simulink model "Ond_MLI_1"  (R2020a)
settings: Solver=VariableStepAuto  StartTime=0.0  StopTime=1  FixedStep=0.0001  RelTol=1e-3  EnableMultiTasking=on
InitFcn:
  | E=150;
  | V=220;
  | fs=50;
  | A=1;
  | 
  | Teta_0=0;
  | Cr=0;
  | Rr=3.805;
  | J=0.031;
  | f=0;
  | p=2;
  | Rs=4.85;
  | M=0.258;
  | Ls=0.274;
  | Lr=0.274;
  | R=[Rs 0 0 0;0 Rs 0 0;0 0 Rs 0;0 0 0 Rs];
  | L=[Ls 0 M 0;0 Ls 0 M;M 0 Lr 0;0 M 0 Lr];
  | A1=[0 -Ls 0 -M;Ls 0 M 0;0 0 0 0;0 0 0 0];
  | A2=[0 0 0 0;0 0 0 0;0 -M 0 -Lr;M 0 Lr 0];
undefined symbols (not defined in the file): Vp
libraries: powerlib x11, simulink x2, powerlib_meascontrol x2
settings Model: SimulationMode=accelerator  Creator=SINA  LastModifiedBy=ABO-CHIFA
settings DataIOCC: ReturnWorkspaceOutputs=off
settings OptimizationCC: LifeSpan=inf
settings DebuggingCC: SFUnexpectedBacktrackingDiag=warning  SFNoUnconditionalDefaultTransitionDiag=warning  ArithmeticOperatorsInVariantConditions=warning
settings SFSimCC: SimUseLocalCustomCode=off  CustomCodeUndefinedFunction=UseInterfaceOnly
settings RTWCC: RTWUseLocalCustomCode=off
settings CodeAppCC: StateflowObjectComments=on
settings GRTTargetCC: TargetLangStandard=C89/C90 (ANSI)
settings ConfigComp: CovMetricSettings=dw  CovHtmlReporting=on  CovSaveCumulativeToWorkspaceVar=on  CovSaveSingleToWorkspaceVar=on  CovExternalEMLEnable=off
settings SimscapeCC: SimscapeNormalizeSystem=off

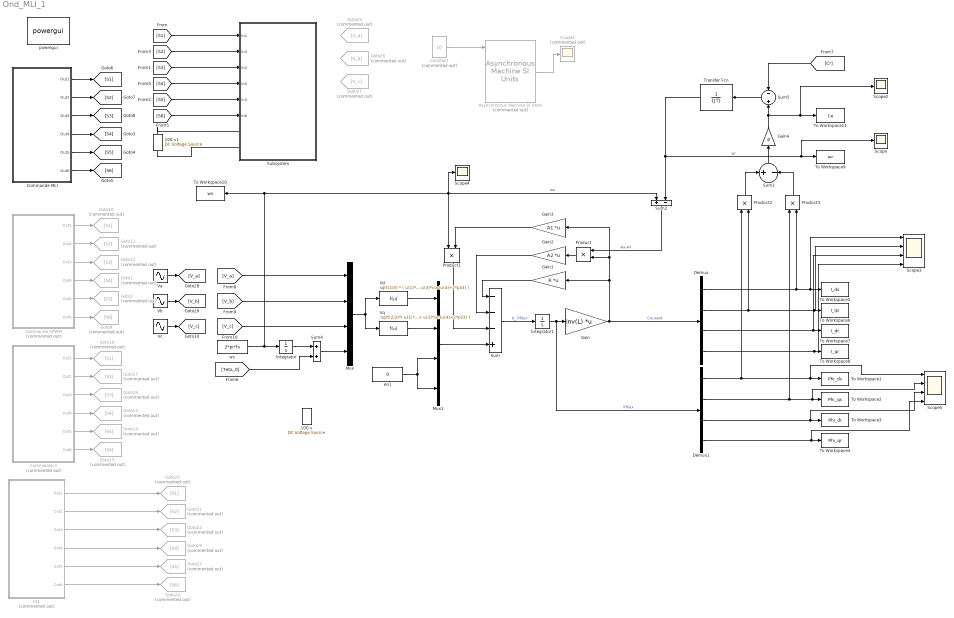
== system Ond_MLI_1 ==
  100 v : powerlib/Electrical Sources/DC Voltage Source  Amplitude=E  Measurements=Voltage
  100 v1 : powerlib/Electrical Sources/DC Voltage Source  Amplitude=E  Measurements=Voltage
  Asynchronous Machine SI Units : powerlib/Machines/Asynchronous Machine SI Units  Commented=on  RotorType=Squirrel-cage  PresetModel="15:  5.4 HP (4KW)   400 V  50Hz 1430 RPM"  MechanicalLoad=Torque Tm  ShowDetailedParameters=on  ReferenceFrame=Rotor  Units=SI  MeasurementBus=off  NominalParameters=[4000 400 50]  Stator=[1.405 0.005839]  Rotor=[1.395 0.005839]  Cage1=[0.4155 0.002066]  Cage2=[0.4168 0.0003495]  Lm=0.1722  Mechanical=[0.0131 0.002985 2]  PolePairs=2  InitialConditions=[1 0 0 0 0 0 0 0]  SimulateSaturation=off  Saturation=[14.03593122, 27.81365428, 53.79336849, 72.68890987, 97.98006896, 148.6815601, 215.7428561, 302.9841135, 428.7778367 ; 230, 322, 414, 460, 506, 552, 598, 644, 690]  LoadFlowParameters=1492000  TsPowergui=0  TsBlock=-1  IterativeModel=Trapezoidal non iterative  IterativeDiscreteModel=Trapezoidal non iterative  Pmec=1.492e+006
  "Commande 3 " : Subsystem  Commented=on
  "Commande MLI " : Subsystem
  "Commande SPWM " : Subsystem  Commented=on
  Constant : Constant  Commented=on  Value=10
  Demux : Demux
  Demux1 : Demux
  Gain : Gain  Gain=inv(L)  Multiplication=Matrix(K*u)
  Gain1 : Gain  Gain=R  Multiplication=Matrix(K*u)
  Gain2 : Gain  Gain=A2  Multiplication=Matrix(K*u)
  Gain3 : Gain  Gain=A1  Multiplication=Matrix(K*u)
  Gain4 : Gain  Gain=p
  Goto1 : Goto  Commented=on  GotoTag=S4
  Goto10 : Goto  Commented=on  GotoTag=S1
  Goto11 : Goto  Commented=on  GotoTag=S2
  Goto12 : Goto  Commented=on  GotoTag=S3
  Goto13 : Goto  Commented=on  GotoTag=S4
  Goto14 : Goto  Commented=on  GotoTag=S5
  Goto15 : Goto  Commented=on  GotoTag=S6
  Goto16 : Goto  Commented=on  GotoTag=S1
  Goto17 : Goto  Commented=on  GotoTag=S2
  Goto18 : Goto  Commented=on  GotoTag=S3
  Goto19 : Goto  Commented=on  GotoTag=S4
  Goto2 : Goto  Commented=on  GotoTag=S5
  Goto20 : Goto  Commented=on  GotoTag=S1
  Goto21 : Goto  Commented=on  GotoTag=S2
  Goto22 : Goto  Commented=on  GotoTag=S3
  Goto23 : Goto  Commented=on  GotoTag=S5
  Goto24 : Goto  Commented=on  GotoTag=S6
  Goto25 : Goto  Commented=on  GotoTag=V_a
  Goto26 : Goto  Commented=on  GotoTag=V_b
  Goto27 : Goto  Commented=on  GotoTag=V_c
  Goto9 : Goto  Commented=on  GotoTag=S6
  Integrator : Integrator
  Integrator1 : Integrator
  Mux : Mux
  Mux1 : Mux
  Product{,1..3} (4 alike) : Product
  Scope : Scope
  Scope1 : Scope  Commented=on
  Scope2 : Scope
  Scope3 : Scope  NumInputPorts=4
  Scope4 : Scope
  Scope5 : Scope  NumInputPorts=4
  Subsystem : Subsystem
  Sum : Sum  Inputs=---+
  Sum1 : Sum  Inputs=+-
  Sum2 : Sum  Inputs=+-
  Sum4 : Sum
  Sum5 : Sum  Inputs=-+
  To Workspace1 : ToWorkspace  VariableName=Phi_ds  SampleTime=-1
  To Workspace10 : ToWorkspace  VariableName=ws  SampleTime=-1
  To Workspace11 : ToWorkspace  VariableName=Ce  SampleTime=-1
  To Workspace2 : ToWorkspace  VariableName=Phi_qs  SampleTime=-1
  To Workspace3 : ToWorkspace  VariableName=Phi_dr  SampleTime=-1
  To Workspace4 : ToWorkspace  VariableName=Phi_qr  SampleTime=-1
  To Workspace5 : ToWorkspace  VariableName=I_ds  SampleTime=-1
  To Workspace6 : ToWorkspace  VariableName=I_qs  SampleTime=-1
  To Workspace7 : ToWorkspace  VariableName=I_dr  SampleTime=-1
  To Workspace8 : ToWorkspace  VariableName=I_qr  SampleTime=-1
  To Workspace9 : ToWorkspace  VariableName=wr  SampleTime=-1
  Transfer Fcn : TransferFcn  Denominator=[J f]
  Va : Sin  Amplitude=V*sqrt(2)  Frequency=2*pi*fs  SampleTime=0
  Vb : Sin  Amplitude=V*sqrt(2)  Frequency=2*pi*fs  Phase=-2*pi/3  SampleTime=0
  Vc : Sin  Amplitude=V*sqrt(2)  Frequency=2*pi*fs  Phase=2*pi/3  SampleTime=0
  Vd : Fcn  Expr="sqrt(2/3) * ( u(1)*cos(u(4))  + u(2)*cos(u(4)-2*pi/3) + u(3)*cos(u(4)+2*pi/3) )"
  Vq : Fcn  Expr="-sqrt(2/3)*( u(1)*sin(u(4))  + u(2)*sin(u(4)-2*pi/3) + u(3)*sin(u(4)+2*pi/3) )"
  powergui : powerlib/powergui  Priority=1  SimulationMode=Discrete  SampleTime=1e-6  frequency=60  Iterations=50  frequencyindice=0  Pbase=100e6  ErrMax=1e-4  UnitsV=kV  UnitsW=MW  buscounter=0  FunctionMessages=off  echomessages=off  EnableUseOfTLC=off  CurrentSourceSwitches=off  DisableSnubberDevices=off  DisableRonSwitches=off  DisableVfSwitches=off  DisplayEquations=off  AutomaticDiscreteSolvers=off  SolverType=Tustin/Backward Euler (TBE)  Interpol=off  ExternalGateDelay=off  methode=off  Ts=10  x0status=blocks  SPID=off  SwTol=0  HookPort=off  NonlinearTolerance=1e-4  nMaxIteration=100  ContinueOnMaxIteration=off  RestoreLinks=warning  ResistiveCurrentMeasurement=off  Frange=[0:2:500]  Ylog=off  Xlog=on  ShowGrid=off  save=off  variable=ZData  structure=0  ZoomFFT=off  StartTime=0.0  cycles=1  DisplayStyle=1  fundamental=60  FreqAxis=off  MaxFrequency=1000  frequencyindicesteady=1  RmsSteady=1  display=off
  "tri1 " : Subsystem  Commented=on
  ws : Constant  Value=2*pi*fs
  ws1 : Constant  Value=0
  wires:
  "Commande MLI "/4(Out4) -> [S4]
  "Commande MLI "/5(Out5) -> [S5]
  "Commande MLI "/6(Out6) -> [S6]
  "Commande MLI "/2(Out2) -> [S2]
  "Commande MLI "/1(Out1) -> [S1]
  "Commande MLI "/3(Out3) -> [S3]
  "Commande SPWM "/1(Out1) -> Goto10/1
  "Commande SPWM "/2(Out2) -> Goto11/1
  "Commande SPWM "/3(Out3) -> Goto12/1
  "Commande SPWM "/4(Out4) -> Goto1/1
  "Commande SPWM "/5(Out5) -> Goto2/1
  "Commande SPWM "/6(Out6) -> Goto9/1
  [S1] -> Subsystem/1(In1)
  [S3] -> Subsystem/3(In2)
  [S5] -> Subsystem/5(In3)
  [S2] -> Subsystem/2(In4)
  [S4] -> Subsystem/4(In5)
  [S6] -> Subsystem/6(In6)
  "Commande 3 "/1(Out1) -> Goto16/1
  "Commande 3 "/2(Out2) -> Goto17/1
  "Commande 3 "/3(Out3) -> Goto18/1
  "Commande 3 "/4(Out4) -> Goto13/1
  "Commande 3 "/5(Out5) -> Goto14/1
  "Commande 3 "/6(Out6) -> Goto15/1
  Asynchronous Machine SI Units/1 -> Scope1/1
  Constant/1 -> Asynchronous Machine SI Units/1
  "tri1 "/1(Out1) -> Goto20/1
  "tri1 "/2(Out2) -> Goto21/1
  "tri1 "/3(Out3) -> Goto22/1
  "tri1 "/4(Out4) -> Goto19/1
  "tri1 "/5(Out5) -> Goto23/1
  "tri1 "/6(Out6) -> Goto24/1
  ws/1 -> Sum2/1, Scope4/1, Product1/1, To Workspace10/1, Integrator/1  "ws"
  Mux/1 -> Vd/1, Vq/1
  Vd/1 -> Mux1/1
  Vq/1 -> Mux1/2
  ws1/1 -> Mux1/3, Mux1/4
  Sum/1 -> Integrator1/1  "d_ Phlux"
  Integrator1/1 -> Gain/1, Demux1/1  "Phlux"
  Gain/1 -> Demux/1, Gain3/1, Product/2, Gain1/1  "Courant"
  Product/1 -> Gain2/1
  Gain3/1 -> Product1/2
  Demux1/1 -> Product2/1, Scope5/1, To Workspace1/1
  Demux1/4 -> Scope5/4, To Workspace4/1
  Demux1/3 -> Scope5/3, To Workspace3/1
  Demux/4 -> Scope3/4, To Workspace8/1
  Demux/3 -> Scope3/3, To Workspace7/1
  Demux/2 -> Scope3/2, To Workspace6/1, Product2/2
  Demux/1 -> Scope3/1, To Workspace5/1, Product3/2
  Demux1/2 -> Product3/1, Scope5/2, To Workspace2/1
  Product2/1 -> Sum1/1
  Product3/1 -> Sum1/2
  Transfer Fcn/1 -> To Workspace9/1, Scope/1, Sum2/2  "wr"
  Sum2/1 -> Product/1  "ws-wr"
  Sum1/1 -> Gain4/1
  Integrator/1 -> Sum4/1
  Sum4/1 -> Mux/4
  [Teta_0] -> Sum4/2
  Sum5/1 -> Transfer Fcn/1
  Gain4/1 -> Sum5/2, To Workspace11/1, Scope2/1
  [V_a] -> Mux/1
  [V_b] -> Mux/2
  Vb/1 -> [V_b]
  Va/1 -> [V_a]
  Vc/1 -> [V_c]
  [V_c] -> Mux/3
  Mux1/1 -> Sum/4
  Product1/1 -> Sum/3
  Gain2/1 -> Sum/2
  Gain1/1 -> Sum/1
  [Cr] -> Sum5/1
  connections:
  100 v1/RConn1 -- Subsystem/LConn1
  100 v1/LConn1 -- Subsystem/LConn2

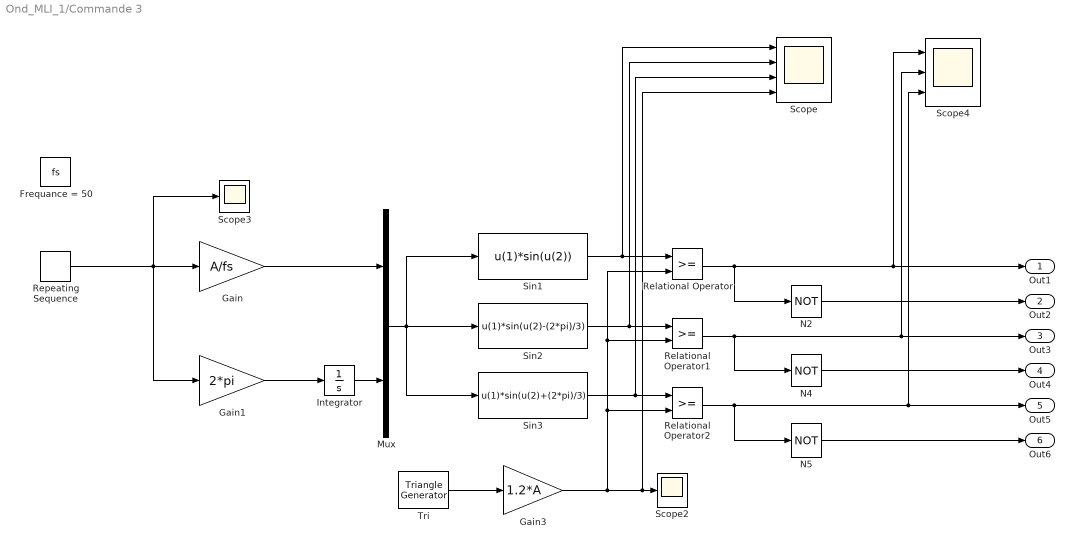
== system Ond_MLI_1/Commande 3  ==
  Frequance = 50 : Constant  Value=fs
  Gain : Gain  Gain=A/fs
  Gain1 : Gain  Gain=2*pi
  Gain3 : Gain  Gain=1.2*A
  Integrator : Integrator
  Mux : Mux  Inputs=2
  N2 : Logic  Operator=NOT  AllPortsSameDT=off  OutDataTypeStr=boolean
  N4 : Logic  Operator=NOT  AllPortsSameDT=off  OutDataTypeStr=boolean
  N5 : Logic  Operator=NOT  AllPortsSameDT=off  OutDataTypeStr=boolean
  Relational Operator : RelationalOperator  OutDataTypeStr=boolean  RndMeth=Nearest
  Relational Operator1 : RelationalOperator  OutDataTypeStr=boolean  RndMeth=Nearest
  Relational Operator2 : RelationalOperator  OutDataTypeStr=boolean  RndMeth=Nearest
  Repeating Sequence : simulink/Sources/Repeating Sequence  rep_seq_t=[0 0.1 10]  rep_seq_y=[0 fs fs]
  Scope : Scope  NumInputPorts=4
  Scope2 : Scope
  Scope3 : Scope
  Scope4 : Scope  NumInputPorts=3
  Sin1 : Fcn  Expr=u(1)*sin(u(2))
  Sin2 : Fcn  Expr=u(1)*sin(u(2)-(2*pi)/3)
  Sin3 : Fcn  Expr=u(1)*sin(u(2)+(2*pi)/3)
  Tri : powerlib_meascontrol/Pulse & Signal Generators/Triangle Generator  Freq=1e3  Phase=90  Ts=0
  Out1 : Outport
  Out2 : Outport  Port=2
  Out3 : Outport  Port=3
  Out4 : Outport  Port=4
  Out5 : Outport  Port=5
  Out6 : Outport  Port=6
  wires:
  Gain1/1 -> Integrator/1
  Integrator/1 -> Mux/2
  Gain/1 -> Mux/1
  Mux/1 -> Sin3/1, Sin2/1, Sin1/1
  N2/1 -> Out2/1
  N4/1 -> Out4/1
  Relational Operator2/1 -> N5/1, Out5/1, Scope4/3
  Gain3/1 -> Relational Operator2/2, Relational Operator1/2, Relational Operator/2, Scope2/1, Scope/4
  Tri/1 -> Gain3/1
  Sin1/1 -> Relational Operator/1, Scope/1
  Sin2/1 -> Relational Operator1/1, Scope/2
  Sin3/1 -> Relational Operator2/1, Scope/3
  N5/1 -> Out6/1
  Relational Operator1/1 -> N4/1, Out3/1, Scope4/2
  Relational Operator/1 -> Out1/1, Scope4/1, N2/1
  Repeating Sequence/1 -> Gain1/1, Scope3/1, Gain/1

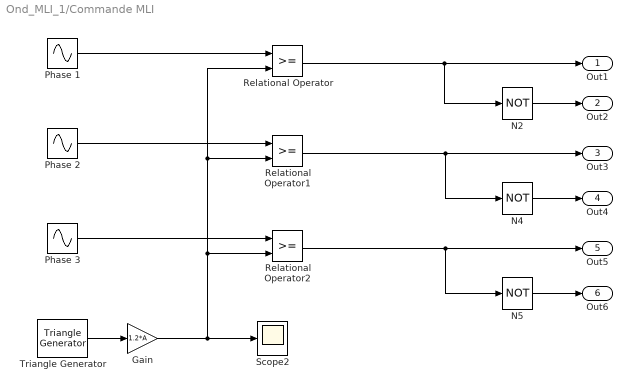
== system Ond_MLI_1/Commande MLI  ==
  Gain : Gain  Gain=1.2*A
  N2 : Logic  Operator=NOT  AllPortsSameDT=off  OutDataTypeStr=boolean
  N4 : Logic  Operator=NOT  AllPortsSameDT=off  OutDataTypeStr=boolean
  N5 : Logic  Operator=NOT  AllPortsSameDT=off  OutDataTypeStr=boolean
  "Phase 1 " : Sin  Amplitude=A  Frequency=2*pi*fs  SampleTime=0
  Phase 2 : Sin  Amplitude=A  Frequency=2*pi*fs  Phase=-2*pi/3  SampleTime=0
  Phase 3 : Sin  Amplitude=A  Frequency=2*pi*fs  Phase=2*pi/3  SampleTime=0
  Relational Operator : RelationalOperator  OutDataTypeStr=boolean  RndMeth=Nearest
  Relational Operator1 : RelationalOperator  OutDataTypeStr=boolean  RndMeth=Nearest
  Relational Operator2 : RelationalOperator  OutDataTypeStr=boolean  RndMeth=Nearest
  Scope2 : Scope
  Triangle Generator : powerlib_meascontrol/Pulse & Signal Generators/Triangle Generator  Freq=1e3  Phase=90  Ts=0
  Out1 : Outport
  Out2 : Outport  Port=2
  Out3 : Outport  Port=3
  Out4 : Outport  Port=4
  Out5 : Outport  Port=5
  Out6 : Outport  Port=6
  wires:
  Phase 3/1 -> Relational Operator2/1
  N4/1 -> Out4/1
  N5/1 -> Out6/1
  N2/1 -> Out2/1
  Relational Operator/1 -> N2/1, Out1/1
  Relational Operator1/1 -> Out3/1, N4/1
  Relational Operator2/1 -> Out5/1, N5/1
  Phase 2/1 -> Relational Operator1/1
  "Phase 1 "/1 -> Relational Operator/1
  Triangle Generator/1 -> Gain/1
  Gain/1 -> Relational Operator2/2, Relational Operator1/2, Relational Operator/2, Scope2/1

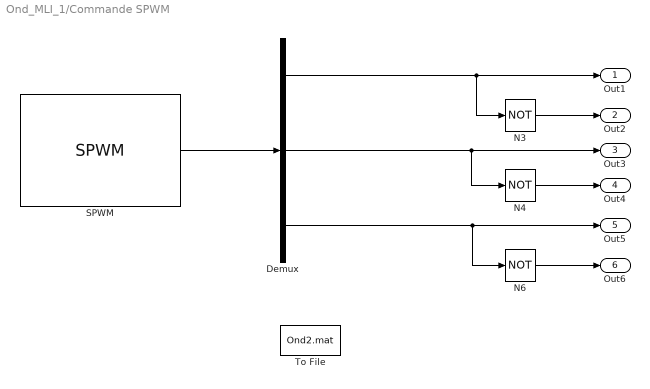
== system Ond_MLI_1/Commande SPWM  ==
  Demux : Demux  Outputs=3
  N3 : Logic  Operator=NOT  AllPortsSameDT=off  OutDataTypeStr=boolean
  N4 : Logic  Operator=NOT  AllPortsSameDT=off  OutDataTypeStr=boolean
  N6 : Logic  Operator=NOT  AllPortsSameDT=off  OutDataTypeStr=boolean
  SPWM : S-Function  FunctionName=SPWM  Parameters=""  SFunctionDeploymentMode=off  EnableBusSupport=off
  To File : ToFile  Filename=Ond2.mat  SaveFormat=Timeseries
  Out1 : Outport
  Out2 : Outport  Port=2
  Out3 : Outport  Port=3
  Out4 : Outport  Port=4
  Out5 : Outport  Port=5
  Out6 : Outport  Port=6
  wires:
  Demux/2 -> Out3/1, N4/1
  N4/1 -> Out4/1
  Demux/1 -> Out1/1, N3/1
  N6/1 -> Out6/1
  N3/1 -> Out2/1
  Demux/3 -> Out5/1, N6/1
  SPWM/1 -> Demux/1

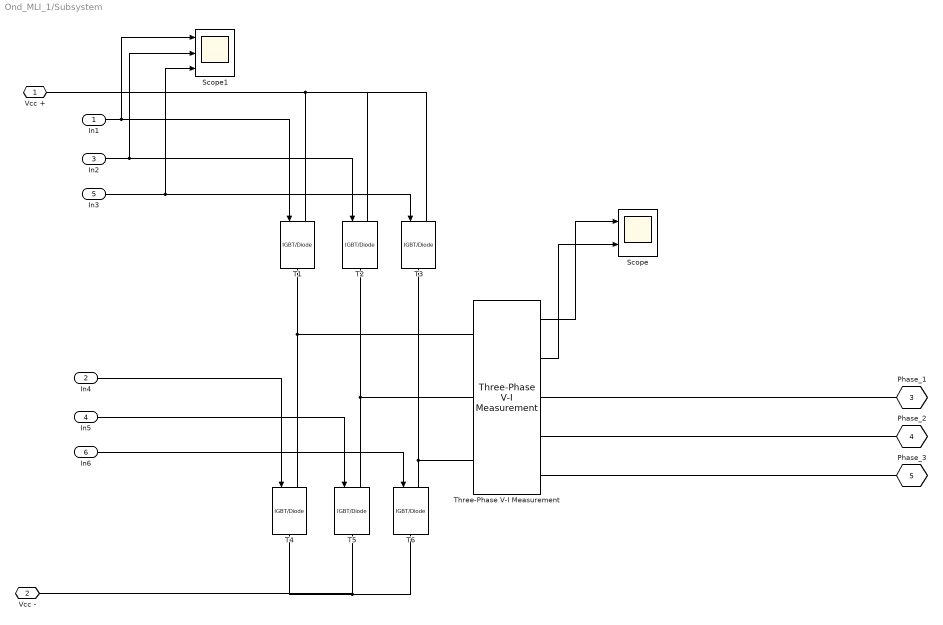
== system Ond_MLI_1/Subsystem ==
  In1 : Inport
  In4 : Inport  Port=2
  In2 : Inport  Port=3
  In5 : Inport  Port=4
  In3 : Inport  Port=5
  In6 : Inport  Port=6
  Scope : Scope  NumInputPorts=2
  Scope1 : Scope  NumInputPorts=3
  T{1..6} (6 alike) : powerlib/Power Electronics/IGBT//Diode  Ron=1e-3  Rs=1e5  Cs=inf  Measurements=off
  Three-Phase V-I Measurement : powerlib/Measurements/Three-Phase V-I Measurement  VoltageMeasurement=phase-to-phase  SetLabelV=off  LabelV=Vabc  Vpu=off  VpuLL=off  CurrentMeasurement=yes  SetLabelI=off  LabelI=Iabc  Ipu=off  Pbase=100e6  Vbase=500e3  OutputType=Complex  PhasorSimulation=off  PSBequivalent=0
  Vcc + : PMIOPort  Side=Left
  Vcc - : PMIOPort  Port=2  Side=Left
  Phase_1 : PMIOPort  Tag=PMCPort  Port=3  Side=Right
  Phase_2 : PMIOPort  Tag=PMCPort  Port=4  Side=Right
  Phase_3 : PMIOPort  Tag=PMCPort  Port=5  Side=Right
  wires:
  Three-Phase V-I Measurement/1 -> Scope/1
  Three-Phase V-I Measurement/2 -> Scope/2
  In1/1 -> Scope1/1, T1/1
  In2/1 -> Scope1/2, T2/1
  In3/1 -> Scope1/3, T3/1
  In4/1 -> T4/1
  In5/1 -> T5/1
  In6/1 -> T6/1
  connections:
  T2/LConn1 -- T3/LConn1 -- Vcc +/RConn1 -- T1/LConn1
  T5/RConn1 -- T4/RConn1 -- Vcc -/RConn1 -- T6/RConn1
  Three-Phase V-I Measurement/LConn1 -- T1/RConn1 -- T4/LConn1
  T5/LConn1 -- T2/RConn1 -- Three-Phase V-I Measurement/LConn2
  T6/LConn1 -- T3/RConn1 -- Three-Phase V-I Measurement/LConn3
  Phase_1/RConn1 -- Three-Phase V-I Measurement/RConn1
  Phase_3/RConn1 -- Three-Phase V-I Measurement/RConn3
  Phase_2/RConn1 -- Three-Phase V-I Measurement/RConn2

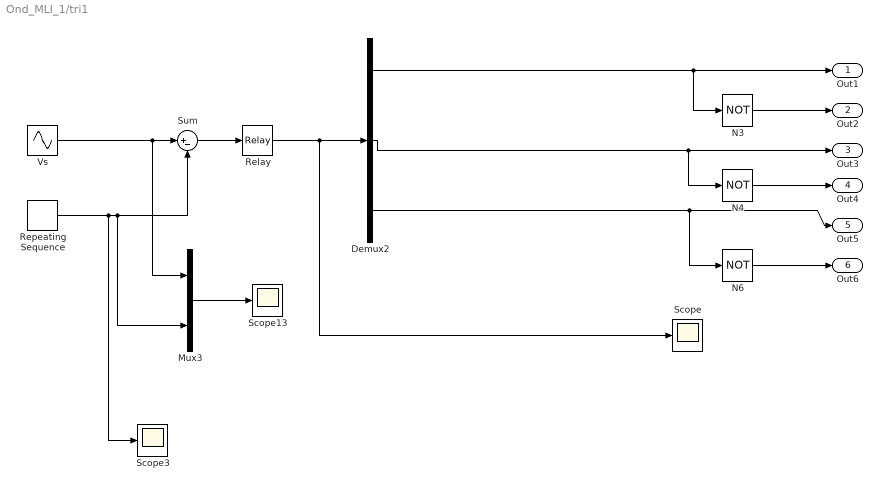
== system Ond_MLI_1/tri1  ==
  Demux2 : Demux  Outputs=3
  Mux3 : Mux  Inputs=2
  N3 : Logic  Operator=NOT  AllPortsSameDT=off  OutDataTypeStr=boolean
  N4 : Logic  Operator=NOT  AllPortsSameDT=off  OutDataTypeStr=boolean
  N6 : Logic  Operator=NOT  AllPortsSameDT=off  OutDataTypeStr=boolean
  Relay : Relay
  Repeating Sequence : simulink/Sources/Repeating Sequence  rep_seq_t="[0 1  2]/5000"  rep_seq_y=[-Vp Vp -Vp]
  Scope : Scope
  Scope13 : Scope
  Scope3 : Scope
  Sum : Sum  Inputs=|+-
  Vs : Sin  Amplitude=A  Frequency=2*pi*fs  Phase=[0 -2*pi/3 2*pi/3]  SampleTime=0
  Out1 : Outport
  Out2 : Outport  Port=2
  Out3 : Outport  Port=3
  Out4 : Outport  Port=4
  Out5 : Outport  Port=5
  Out6 : Outport  Port=6
  wires:
  Vs/1 -> Sum/1, Mux3/1
  Repeating Sequence/1 -> Scope3/1, Sum/2, Mux3/2
  Sum/1 -> Relay/1
  Mux3/1 -> Scope13/1
  N3/1 -> Out2/1
  Demux2/3 -> N6/1, Out5/1
  Demux2/1 -> N3/1, Out1/1
  N4/1 -> Out4/1
  N6/1 -> Out6/1
  Relay/1 -> Scope/1, Demux2/1
  Demux2/2 -> Out3/1, N4/1
